simulink model "M_6DoF_BS_Full_backup_11_25_2018"  (R2018a)
settings: Solver=ode4  StartTime=0.0  StopTime=80  FixedStep=0.01  RelTol=1e-3  EnableMultiTasking=on
values from neighbouring files (symbols this model uses):
  b = 1.5652e-08 * (60/(2*pi))^2    (= 1.42729124973e-06)    [Main_run.m]    (also in golden_search.m = x2)
  cbar = 0.04    [Main_run.m]
  Cd = 0.001    [Main_run.m]
  deltaT = 15    [Main_run.m]
  g = 9.81    [Main_run.m]
  Gama1 = diag([3,3,3])    [Main_run.m]
  Gama2 = diag([0.1,0.1,0.1])    [Main_run.m]
  I_B = diag([Ix,Iy,Iz])    [Main_run.m]
  I_r = 3.357e-5    (= 3.357e-05)    [Main_run.m]
  InitialEulerAngles = [psi_i,theta_i,phi_i]    [Main_run.m]
  k = 2.0862e-10 * (60/(2*pi))^2    (= 1.90238627983e-08)    [Main_run.m]    (also in golden_search.m = 2)
  Kd = diag([2,2,2])    [Main_run.m]
  Ki = diag([0.01,0.01,0.01])    [Main_run.m]
  Kp = diag([1,1,1])    [Main_run.m]
  l = 0.225    [Main_run.m]    (also in try1.m = nb * trapz(psi, cl * 0.5 .* rho .* (vt*u).^2 .*c2 , 2) / (2*; try2.m = nb * trapz(psi, cl * 0.5 .* rho .* (vt*u).^2 .*c2 , 2) / (2*)
  Lambda = diag([10,10,10])    [Main_run.m]
  m = 1.035 * 4/6    (= 0.69)    [Main_run.m]
  Omega_i = [0;0;0]    [Main_run.m]
  r = linspace(floor(nr*0.01)/nr,1,nr)    [Main_run.m]    (also in Propeller.m = geometry(10,1:nr); try1.m = geometry(10,1:nr); try2.m = geometry(10,1:nr))
  R_i = [0.0;0.0;0.0]    [Main_run.m]
  t_phase3 = 10    [Main_run.m]
  Tbar = diag([15,15,15])    [Main_run.m]
  tf_phase1 = 10    [Main_run.m]
  tf_phase2 = tf_phase1 + length_phase2*60    (= 70)    [Main_run.m]
  V_i = [0.0;0.0;-0.001]    [Main_run.m]
  Wind_dir = 30 + 180    (= 210)    [Main_run.m]
  xdot_cruise = 15    [Main_run.m]
  zf_phase1 = -40    [Main_run.m]
undefined symbols (not defined in the file or in its folder): eul_0, HDBK, MIL, Moderate, wind_table, wind_time
libraries: sharedtransform x6, aerolibconvert2 x3, aerolibwind2 x3, sharedutil x2, simulink x1, aerolibutil x1, dspmathops x1
(part 1 of 2)
settings Model: SimulationMode=accelerator  Creator=EhsanTaheri  LastModifiedBy=behdad
settings SolverCC: AlgebraicLoopSolver=LineSearch
settings DataIOCC: LimitDataPoints=on  SaveFormat=Array
settings OptimizationCC: EfficientMapNaN2IntZero=off  LifeSpan=inf
settings DebuggingCC: SolverPrmCheckMsg=warning  SFUnexpectedBacktrackingDiag=warning  SFNoUnconditionalDefaultTransitionDiag=warning  SFExecutionAtInitializationDiag=none
settings HardwareCC: ProdBitPerPointer=32  ProdBitPerSizeT=32  ProdBitPerPtrDiffT=32  ProdLargestAtomicFloat=None  ProdIntDivRoundTo=Undefined  ProdEndianess=Unspecified  ProdWordSize=32  ProdHWDeviceType=32-bit Generic  TargetBitPerLong=64  TargetBitPerPointer=64  TargetBitPerSizeT=64  TargetBitPerPtrDiffT=64  TargetLongLongMode=on  TargetIntDivRoundTo=Zero  TargetEndianess=LittleEndian  TargetWordSize=64  TargetHWDeviceType=MATLAB Host  ProdEqTarget=off
settings ModelReferenceCC: PropagateSignalLabelsOutOfModel=off
settings CodeAppCC: MaxIdLength=128
settings GRTTargetCC: TargetLangStandard=C89/C90 (ANSI)  CombineOutputUpdateFcns=off  GRTInterface=on
settings ConfigComp: CovMetricSettings=dw  CovHtmlReporting=on  CovSaveCumulativeToWorkspaceVar=on  CovSaveSingleToWorkspaceVar=on  CovExternalEMLEnable=off  CovSFcnEnable=off

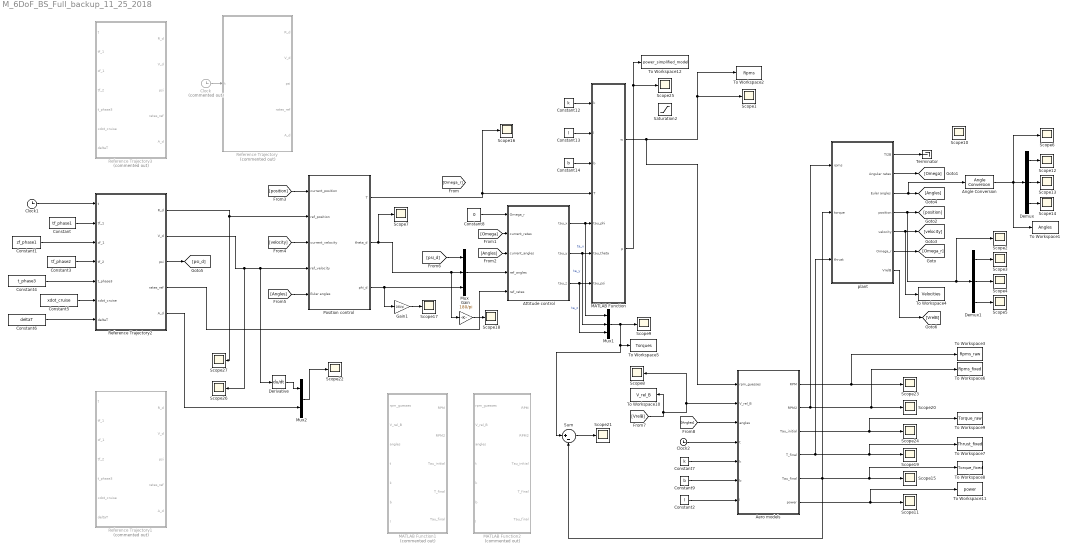
== system M_6DoF_BS_Full_backup_11_25_2018 ==
  Aero models : Subsystem
  Angle Conversion : aerolibconvert2/Angle Conversion  IU=rad  OU=deg
  Attitude control : Subsystem
  Clock : Clock  Commented=on
  Clock1 : Clock
  Clock2 : Clock
  Constant : Constant  Value=tf_phase1
  Constant1 : Constant  Value=zf_phase1
  Constant12 : Constant  Value=k
  Constant13 : Constant  Value=l
  Constant14 : Constant  Value=b
  Constant2 : Constant  Value=l
  Constant3 : Constant  Value=tf_phase2
  Constant4 : Constant  Value=t_phase3
  Constant5 : Constant  Value=xdot_cruise
  Constant6 : Constant  Value=deltaT
  Constant7 : Constant  Value=k
  Constant8 : Constant  Value=0
  Constant9 : Constant  Value=b
  Demux : Demux  Outputs=3
  Demux1 : Demux  Outputs=3
  Derivative : Derivative
  Gain : Gain  Gain=180/pi
  Gain1 : Gain  Gain=180/pi
  MATLAB Function : MATLAB Function  TreatAsAtomicUnit=on
  MATLAB Function1 : MATLAB Function  Commented=on  TreatAsAtomicUnit=on
  MATLAB Function2 : MATLAB Function  Commented=on  TreatAsAtomicUnit=on
  Mux : Mux  Inputs=3
  Mux1 : Mux  Inputs=3
  Mux2 : Mux  Inputs=2
  Position control : Subsystem
  Reference Trajectory : MATLAB Function  Commented=on  TreatAsAtomicUnit=on
  Reference Trajectory1 : MATLAB Function  Commented=on  TreatAsAtomicUnit=on
  Reference Trajectory2 : MATLAB Function  TreatAsAtomicUnit=on
  Reference Trajectory3 : MATLAB Function  Commented=on  TreatAsAtomicUnit=on
  Saturation2 : Saturate  UpperLimit=850  LowerLimit=200
  Scope{1..27} (27 alike) : Scope
  Sum : Sum  Inputs=|+-
  Terminator : Terminator
  To Workspace1 : ToWorkspace  VariableName=Angles  SampleTime=-1
  To Workspace10 : ToWorkspace  VariableName=V_rel_B  SampleTime=-1
  To Workspace11 : ToWorkspace  VariableName=power  SampleTime=-1
  To Workspace12 : ToWorkspace  VariableName=power_simplified_model  SampleTime=-1
  To Workspace2 : ToWorkspace  VariableName=Rpms  SampleTime=-1
  To Workspace3 : ToWorkspace  VariableName=Rpms_raw  SampleTime=-1
  To Workspace4 : ToWorkspace  VariableName=Velocities  SaveFormat=Structure With Time  SampleTime=-1
  To Workspace5 : ToWorkspace  VariableName=Torques  SampleTime=-1
  To Workspace6 : ToWorkspace  VariableName=Rpms_fixed  SampleTime=-1
  To Workspace7 : ToWorkspace  VariableName=Thrust_fixed  SampleTime=-1
  To Workspace8 : ToWorkspace  VariableName=Torque_fixed  SampleTime=-1
  To Workspace9 : ToWorkspace  VariableName=Torque_raw  SampleTime=-1
  plant : Subsystem
  wires:
  Demux/3 -> Scope14/1
  Demux/2 -> Scope13/1
  Demux/1 -> Scope12/1
  Demux1/3 -> Scope5/1
  Demux1/2 -> Scope4/1
  Demux1/1 -> Scope3/1
  Angle Conversion/1 -> Scope6/1, To Workspace1/1, Demux/1
  Constant12/1 -> MATLAB Function/1(k)
  Constant13/1 -> MATLAB Function/2(l)
  Constant14/1 -> MATLAB Function/3(b)
  plant/1(TI2B) -> Terminator/1
  plant/6(Omega_r) -> [Omega_r]
  plant/2(Angular rates) -> [Omega]
  [Omega] -> Attitude control/2(current_rates)
  plant/5(velocity) -> [velocity], To Workspace4/1
  [Angles] -> Attitude control/3(current_angles)
  Position control/1(T) -> Scope16/1, MATLAB Function/4(T)
  Attitude control/1(tau_x) -> Mux1/1, MATLAB Function/5(tau_phi)  "ta_x"
  Attitude control/2(tau_y) -> Mux1/2, MATLAB Function/6(tau_theta)  "ta_y"
  Attitude control/3(tau_z) -> Mux1/3, MATLAB Function/7(tau_psi)  "ta_z"
  [position] -> Position control/1(current_position)
  [velocity] -> Position control/3(current_velocity)
  Position control/2(theta_d) -> Scope7/1, Gain/1, Mux/2
  Position control/3(phi_d) -> Gain1/1, Mux/3
  Mux/1 -> Attitude control/4(ref_angles)
  plant/3(Euler angles) -> Angle Conversion/1, [Angles]
  Reference Trajectory2/3(psi) -> [psi_d]
  [psi_d] -> Mux/1
  Reference Trajectory2/1(R_d) -> Scope27/1, Position control/2(ref_position)
  [Angles] -> Position control/5(Euler angles)
  plant/4(position) -> [position], Scope2/1, Demux1/1
  Gain/1 -> Scope18/1
  Reference Trajectory2/5(A_d) -> Mux2/2
  Reference Trajectory2/2(V_d) -> Scope26/1, Derivative/1, Position control/4(ref_velocity)
  Derivative/1 -> Mux2/1
  Mux2/1 -> Scope22/1
  Gain1/1 -> Scope17/1
  Reference Trajectory2/4(rates_ref) -> Attitude control/5(ref_rates)
  Constant8/1 -> Attitude control/1(Omega_r)
  Clock/1 -> Reference Trajectory/1(t)
  Constant6/1 -> Reference Trajectory2/7(deltaT)
  Constant4/1 -> Reference Trajectory2/5(t_phase3)
  Clock1/1 -> Reference Trajectory2/1(t)
  Constant5/1 -> Reference Trajectory2/6(xdot_cruise)
  Constant1/1 -> Reference Trajectory2/3(zf_1)
  Constant3/1 -> Reference Trajectory2/4(tf_2)
  Constant/1 -> Reference Trajectory2/2(tf_1)
  MATLAB Function/1(w) -> Aero models/1(rpm_guesses), To Workspace2/1, Scope1/1
  Constant9/1 -> Aero models/6(b)
  Sum/1 -> Scope21/1
  [VrelB] -> Scope8/1, Aero models/2(V_rel_B), To Workspace10/1
  Constant7/1 -> Aero models/5(k)
  Constant2/1 -> Aero models/7(l)
  Mux1/1 -> Sum/1, To Workspace5/1, Scope9/1
  [Angles] -> Aero models/3(angles)
  Clock2/1 -> Aero models/4(t)
  Aero models/5(Tau_final) -> plant/2("torque "), To Workspace8/1, Scope15/1, Sum/2
  Aero models/3(Tau_initial) -> To Workspace9/1, Scope24/1
  Aero models/2(RPM2) -> Scope20/1, To Workspace6/1, plant/1(rpms)
  Aero models/1(RPM) -> Scope23/1, To Workspace3/1
  Aero models/4(T_final) -> plant/3(thrust), To Workspace7/1, Scope19/1
  plant/7(VrelB) -> [VrelB]
  Aero models/6(power) -> To Workspace11/1, Scope11/1
  MATLAB Function/2(p) -> Scope25/1, To Workspace12/1

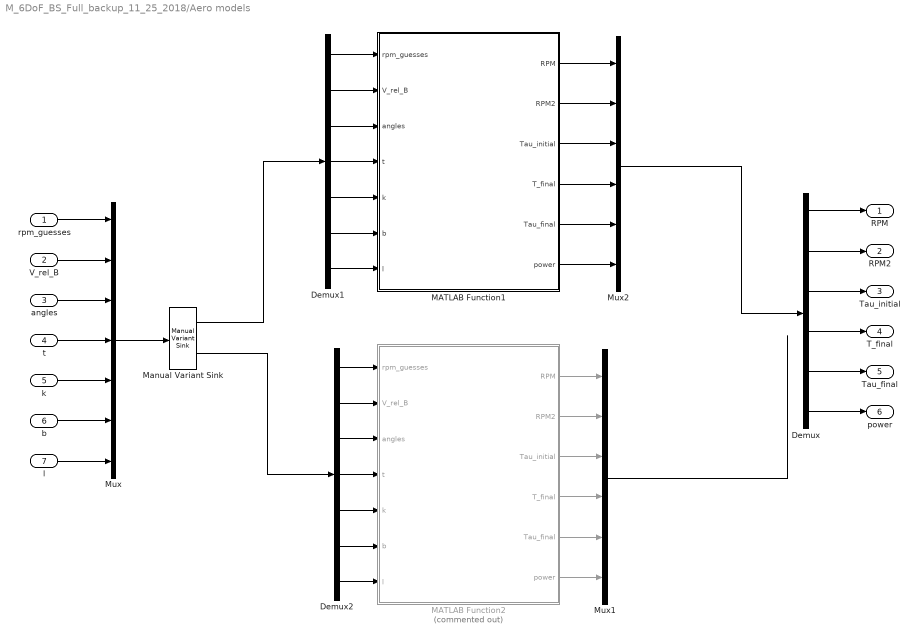
== system M_6DoF_BS_Full_backup_11_25_2018/Aero models ==
  rpm_guesses : Inport
  V_rel_B : Inport  Port=2
  angles : Inport  Port=3
  t : Inport  Port=4
  k : Inport  Port=5
  b : Inport  Port=6
  l : Inport  Port=7
  Demux : Demux  Outputs=[4 4 3 1 3 1]
  Demux1 : Demux  Outputs=[4 3 3 1 1 1 1]
  Demux2 : Demux  Outputs=[4 3 3 1 1 1 1]
  MATLAB Function1 : MATLAB Function  TreatAsAtomicUnit=on
  MATLAB Function2 : MATLAB Function  Commented=on  TreatAsAtomicUnit=on
  Manual Variant Sink : simulink/Signal Routing/Manual Variant Sink  NumChoices=2  OverrideUsingVariant=V_1
      settings: SourceProductName=Simulink
  Mux : Mux  Inputs=7
  Mux1 : Mux  Inputs=6
  Mux2 : Mux  Inputs=6
  RPM : Outport
  RPM2 : Outport  Port=2
  Tau_initial : Outport  Port=3
  T_final : Outport  Port=4
  Tau_final : Outport  Port=5
  power : Outport  Port=6
  wires:
  rpm_guesses/1 -> Mux/1
  V_rel_B/1 -> Mux/2
  angles/1 -> Mux/3
  t/1 -> Mux/4
  k/1 -> Mux/5
  b/1 -> Mux/6
  l/1 -> Mux/7
  Demux/3 -> Tau_initial/1
  Demux/4 -> T_final/1
  Demux/5 -> Tau_final/1
  Demux/2 -> RPM2/1
  Demux/1 -> RPM/1
  MATLAB Function2/5(Tau_final) -> Mux1/5
  MATLAB Function2/4(T_final) -> Mux1/4
  MATLAB Function2/3(Tau_initial) -> Mux1/3
  MATLAB Function2/2(RPM2) -> Mux1/2
  MATLAB Function2/1(RPM) -> Mux1/1
  MATLAB Function1/5(Tau_final) -> Mux2/5
  MATLAB Function1/4(T_final) -> Mux2/4
  MATLAB Function1/3(Tau_initial) -> Mux2/3
  MATLAB Function1/2(RPM2) -> Mux2/2
  MATLAB Function1/1(RPM) -> Mux2/1
  Demux1/7 -> MATLAB Function1/7(l)
  Demux1/6 -> MATLAB Function1/6(b)
  Demux1/5 -> MATLAB Function1/5(k)
  Demux1/4 -> MATLAB Function1/4(t)
  Demux1/3 -> MATLAB Function1/3(angles)
  Demux1/2 -> MATLAB Function1/2(V_rel_B)
  Demux1/1 -> MATLAB Function1/1(rpm_guesses)
  Demux2/7 -> MATLAB Function2/7(l)
  Demux2/6 -> MATLAB Function2/6(b)
  Demux2/5 -> MATLAB Function2/5(k)
  Demux2/4 -> MATLAB Function2/4(t)
  Demux2/3 -> MATLAB Function2/3(angles)
  Demux2/2 -> MATLAB Function2/2(V_rel_B)
  Demux2/1 -> MATLAB Function2/1(rpm_guesses)
  Mux/1 -> Manual Variant Sink/1
  Manual Variant Sink/1 -> Demux1/1
  Manual Variant Sink/2 -> Demux2/1
  MATLAB Function2/6(power) -> Mux1/6
  Demux/6 -> power/1
  MATLAB Function1/6(power) -> Mux2/6
  Mux1/1 -> ?
  Mux2/1 -> Demux/1

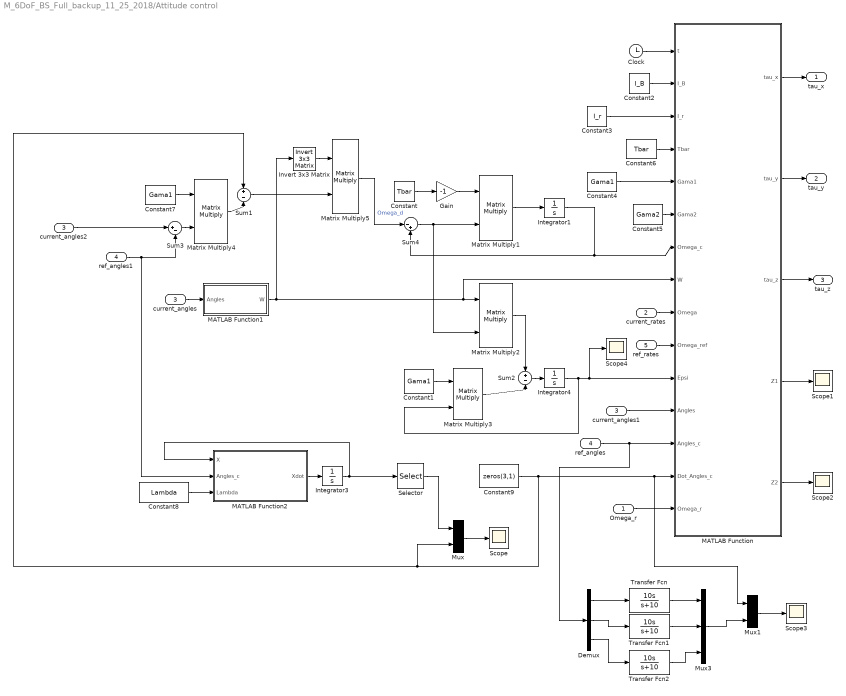
== system M_6DoF_BS_Full_backup_11_25_2018/Attitude control ==
  Omega_r : Inport
  current_rates : Inport  Port=2
  current_angles : Inport  Port=3
  ref_angles : Inport  Port=4
  ref_rates : Inport  Port=5
  Clock : Clock
  Constant : Constant  Value=Tbar
  Constant1 : Constant  Value=Gama1
  Constant2 : Constant  Value=I_B
  Constant3 : Constant  Value=I_r
  Constant4 : Constant  Value=Gama1
  Constant5 : Constant  Value=Gama2
  Constant6 : Constant  Value=Tbar
  Constant7 : Constant  Value=Gama1
  Constant8 : Constant  Value=Lambda
  Constant9 : Constant  Value=zeros(3,1)
  Demux : Demux  Outputs=3
  Gain : Gain  Gain=-1
  Integrator1 : Integrator  InitialCondition=zeros(3,1)
  Integrator3 : Integrator  InitialCondition=[InitialEulerAngles';zeros(3,1)]
  Integrator4 : Integrator  InitialCondition=zeros(3,1)
  Invert 3x3 Matrix : aerolibutil/Invert  3x3 Matrix
  MATLAB Function : MATLAB Function  TreatAsAtomicUnit=on
  MATLAB Function1 : MATLAB Function  TreatAsAtomicUnit=on
  MATLAB Function2 : MATLAB Function  TreatAsAtomicUnit=on
  Matrix Multiply{1..5} (5 alike) : Product  Multiplication=Matrix(*)
  Mux : Mux  Inputs=2
  Mux1 : Mux  Inputs=2
  Mux3 : Mux  Inputs=3
  Scope{,1..4} (5 alike) : Scope
  Selector : Selector  InputPortWidth=6  IndexOptions=Index vector (dialog)  Indices=[4 5 6]  OutputSizes=1
  Sum1 : Sum  Inputs=+|-
  Sum2 : Sum  Inputs=+|-
  Sum3 : Sum  Inputs=|+-
  Sum4 : Sum  Inputs=|-+
  Transfer Fcn : TransferFcn  Numerator=[10 0]  Denominator=[1 10]
  Transfer Fcn1 : TransferFcn  Numerator=[10 0]  Denominator=[1 10]
  Transfer Fcn2 : TransferFcn  Numerator=[10 0]  Denominator=[1 10]
  current_angles1 : InportShadow  Port=3
  current_angles2 : InportShadow  Port=3
  ref_angles1 : InportShadow  Port=4
  tau_x : Outport
  tau_y : Outport  Port=2
  tau_z : Outport  Port=3
  wires:
  Omega_r/1 -> MATLAB Function/15(Omega_r)
  MATLAB Function/1(tau_x) -> tau_x/1
  MATLAB Function/2(tau_y) -> tau_y/1
  MATLAB Function/3(tau_z) -> tau_z/1
  Matrix Multiply5/1 -> Sum4/1  "Omega_d"
  Gain/1 -> Matrix Multiply1/1
  Constant/1 -> Gain/1
  current_angles/1 -> MATLAB Function1/1(Angles)
  MATLAB Function1/1(W) -> Invert 3x3 Matrix/1, MATLAB Function/8(W), Matrix Multiply2/1
  Matrix Multiply1/1 -> Integrator1/1
  Matrix Multiply2/1 -> Sum2/1
  Matrix Multiply3/1 -> Sum2/2
  Constant1/1 -> Matrix Multiply3/1
  Integrator4/1 -> Matrix Multiply3/2, Scope4/1, MATLAB Function/11(Epsi)
  current_rates/1 -> MATLAB Function/9(Omega)
  current_angles1/1 -> MATLAB Function/12(Angles)
  ref_angles/1 -> Demux/1, MATLAB Function/13(Angles_c)
  Constant4/1 -> MATLAB Function/5(Gama1)
  Constant5/1 -> MATLAB Function/6(Gama2)
  Constant6/1 -> MATLAB Function/4(Tbar)
  Constant2/1 -> MATLAB Function/2(I_B)
  Constant3/1 -> MATLAB Function/3(I_r)
  Constant7/1 -> Matrix Multiply4/1
  Sum3/1 -> Matrix Multiply4/2
  current_angles2/1 -> Sum3/1
  ref_angles1/1 -> MATLAB Function2/2(Angles_c), Sum3/2
  Matrix Multiply4/1 -> Sum1/2
  Invert 3x3 Matrix/1 -> Matrix Multiply5/1
  Sum1/1 -> Matrix Multiply5/2
  Integrator1/1 -> Sum4/2, MATLAB Function/7(Omega_c)
  Sum4/1 -> Matrix Multiply2/2, Matrix Multiply1/2
  Clock/1 -> MATLAB Function/1(t)
  MATLAB Function2/1(Xdot) -> Integrator3/1
  Integrator3/1 -> Selector/1, MATLAB Function2/1(X)
  Constant8/1 -> MATLAB Function2/3(Lambda)
  ref_rates/1 -> MATLAB Function/10(Omega_ref)
  Constant9/1 -> Mux/2, Sum1/1, Mux1/1, MATLAB Function/14(Dot_Angles_c)
  Selector/1 -> Mux/1
  MATLAB Function/4(Z1) -> Scope1/1
  MATLAB Function/5(Z2) -> Scope2/1
  Demux/1 -> Transfer Fcn/1
  Demux/2 -> Transfer Fcn1/1
  Demux/3 -> Transfer Fcn2/1
  Transfer Fcn1/1 -> Mux3/2
  Mux3/1 -> Mux1/2
  Mux1/1 -> Scope3/1
  Mux/1 -> Scope/1
  Sum2/1 -> Integrator4/1
  Transfer Fcn/1 -> Mux3/1
  Transfer Fcn2/1 -> Mux3/3

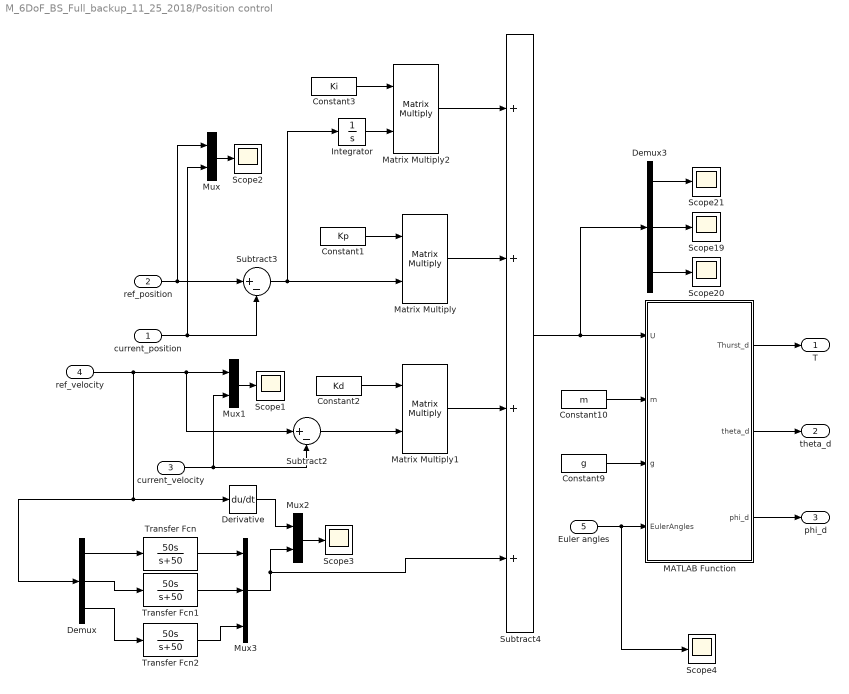
== system M_6DoF_BS_Full_backup_11_25_2018/Position control ==
  current_position : Inport
  ref_position : Inport  Port=2
  current_velocity : Inport  Port=3
  ref_velocity : Inport  Port=4
  Euler angles : Inport  Port=5
  Constant1 : Constant  Value=Kp
  Constant10 : Constant  Value=m
  Constant2 : Constant  Value=Kd
  Constant3 : Constant  Value=Ki
  Constant9 : Constant  Value=g
  Demux : Demux  Outputs=3
  Demux3 : Demux  Outputs=3
  Derivative : Derivative
  Integrator : Integrator  InitialCondition=zeros(3,1)
  MATLAB Function : MATLAB Function  TreatAsAtomicUnit=on
  Matrix Multiply : Product  Multiplication=Matrix(*)
  Matrix Multiply1 : Product  Multiplication=Matrix(*)
  Matrix Multiply2 : Product  Multiplication=Matrix(*)
  Mux : Mux  Inputs=2
  Mux1 : Mux  Inputs=2
  Mux2 : Mux  Inputs=2
  Mux3 : Mux  Inputs=3
  Scope{1..4,19..21} (7 alike) : Scope
  Subtract2 : Sum  Inputs=|+-
  Subtract3 : Sum  Inputs=|+-
  Subtract4 : Sum  Inputs=++++
  Transfer Fcn : TransferFcn  Numerator=[50 0]  Denominator=[1 50]
  Transfer Fcn1 : TransferFcn  Numerator=[50 0]  Denominator=[1 50]
  Transfer Fcn2 : TransferFcn  Numerator=[50 0]  Denominator=[1 50]
  T : Outport
  theta_d : Outport  Port=2
  phi_d : Outport  Port=3
  wires:
  MATLAB Function/2(theta_d) -> theta_d/1
  MATLAB Function/3(phi_d) -> phi_d/1
  MATLAB Function/1(Thurst_d) -> T/1
  Constant10/1 -> MATLAB Function/2(m)
  Constant9/1 -> MATLAB Function/3(g)
  ref_position/1 -> Subtract3/1, Mux/1
  current_position/1 -> Subtract3/2, Mux/2
  Subtract3/1 -> Matrix Multiply/2, Integrator/1
  Constant1/1 -> Matrix Multiply/1
  Subtract2/1 -> Matrix Multiply1/2
  Constant2/1 -> Matrix Multiply1/1
  Subtract4/1 -> Demux3/1, MATLAB Function/1(U)
  Euler angles/1 -> Scope4/1, MATLAB Function/4(EulerAngles)
  Mux/1 -> Scope2/1
  Mux1/1 -> Scope1/1
  Derivative/1 -> Mux2/1
  Mux2/1 -> Scope3/1
  Demux/1 -> Transfer Fcn/1
  Demux/2 -> Transfer Fcn1/1
  Demux/3 -> Transfer Fcn2/1
  Transfer Fcn1/1 -> Mux3/2
  Mux3/1 -> Subtract4/4, Mux2/2
  Integrator/1 -> Matrix Multiply2/2
  Constant3/1 -> Matrix Multiply2/1
  Matrix Multiply1/1 -> Subtract4/3
  Matrix Multiply/1 -> Subtract4/2
  Matrix Multiply2/1 -> Subtract4/1
  Transfer Fcn/1 -> Mux3/1
  Transfer Fcn2/1 -> Mux3/3
  current_velocity/1 -> Subtract2/2, Mux1/2
  Demux3/3 -> Scope20/1
  Demux3/1 -> Scope21/1
  Demux3/2 -> Scope19/1
  ref_velocity/1 -> Derivative/1, Demux/1, Mux1/1, Subtract2/1

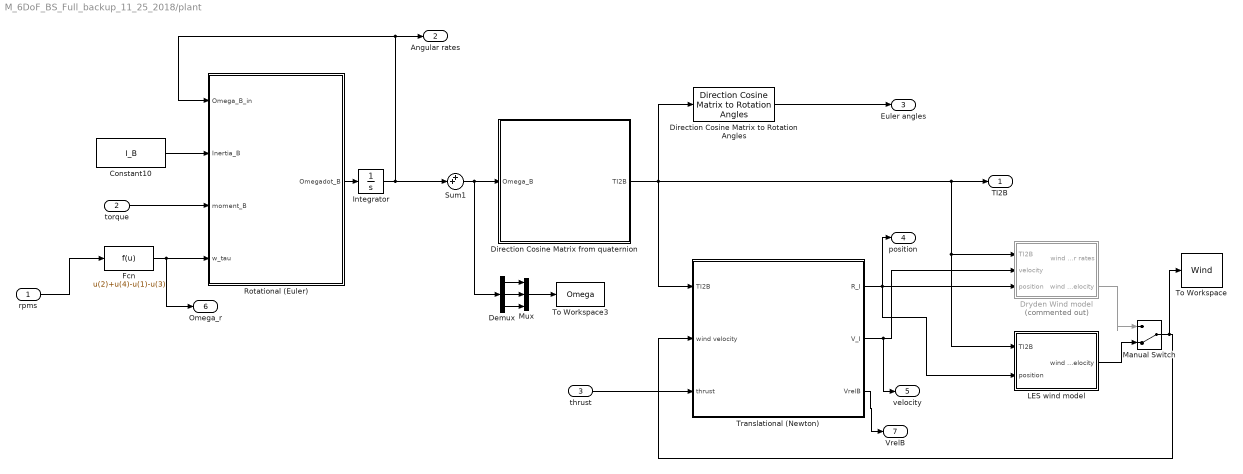
== system M_6DoF_BS_Full_backup_11_25_2018/plant ==
  rpms : Inport
  "torque " : Inport  Port=2
  thrust : Inport  Port=3
  Constant10 : Constant  Value=I_B
  Demux : Demux  Outputs=3
  Direction Cosine Matrix to Rotation Angles : sharedtransform/Direction Cosine Matrix to Rotation Angles  rotationOrder=ZYX  aMode=aMode  action=None  tolerance=eps(2)
      settings: SourceProductName=Aerospace Blockset  SourceProductBaseCode=AE
  Direction Cosine Matrix from quaternion : Subsystem
  Dryden Wind model : Subsystem  Commented=on
  Fcn : Fcn  Expr=u(2)+u(4)-u(1)-u(3)
  Integrator : Integrator  InitialCondition=Omega_i
  LES wind model : Subsystem
  Manual Switch : ManualSwitch  CurrentSetting=0
  Mux : Mux  Inputs=3
  Rotational (Euler) : Subsystem
  Sum1 : Sum  Inputs=++|
  To Workspace : ToWorkspace  VariableName=Wind  SampleTime=-1
      settings: Save2DSignal=2-D array (concatenate along first dimension)
  To Workspace3 : ToWorkspace  VariableName=Omega  SampleTime=-1
  Translational (Newton) : Subsystem
  TI2B : Outport
  Angular rates : Outport  Port=2
  Euler angles : Outport  Port=3
  position : Outport  Port=4
  velocity : Outport  Port=5
  Omega_r : Outport  Port=6
  VrelB : Outport  Port=7
  wires:
  Translational (Newton)/2(V_I) -> velocity/1, Dryden Wind model/2(velocity)
  Direction Cosine Matrix to Rotation Angles/1 -> Euler angles/1
  Constant10/1 -> Rotational (Euler)/2(Inertia_B)
  Rotational (Euler)/1(Omegadot_B) -> Integrator/1
  Direction Cosine Matrix from quaternion/1(TI2B) -> Translational (Newton)/1(TI2B), LES wind model/1(TI2B), Dryden Wind model/1(TI2B), TI2B/1, Direction Cosine Matrix to Rotation Angles/1
  rpms/1 -> Fcn/1
  Fcn/1 -> Rotational (Euler)/4(w_tau), Omega_r/1
  Integrator/1 -> Sum1/2, Angular rates/1, Rotational (Euler)/1(Omega_B_in)
  Sum1/1 -> Demux/1, Direction Cosine Matrix from quaternion/1(Omega_B)
  Demux/1 -> Mux/1
  Demux/2 -> Mux/2
  Demux/3 -> Mux/3
  Mux/1 -> To Workspace3/1
  thrust/1 -> Translational (Newton)/3(thrust)
  "torque "/1 -> Rotational (Euler)/3(moment_B)
  Translational (Newton)/3(VrelB) -> VrelB/1
  Translational (Newton)/1(R_I) -> Dryden Wind model/3(position), LES wind model/2(position), position/1
  LES wind model/1(wind velocity) -> Manual Switch/2
  Dryden Wind model/2(wind velocity) -> Manual Switch/1
  Manual Switch/1 -> To Workspace/1, Translational (Newton)/2(wind velocity)

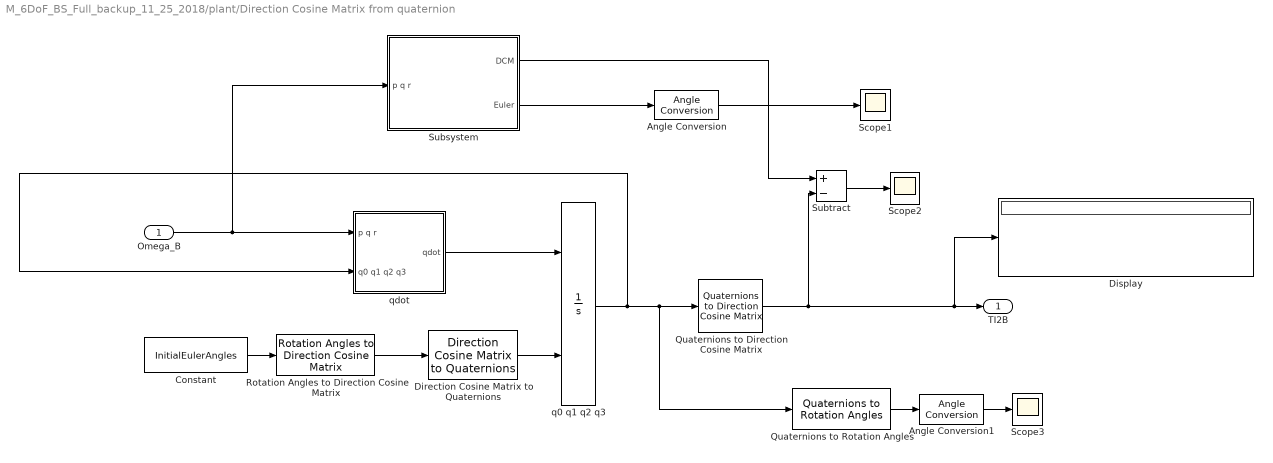
== system M_6DoF_BS_Full_backup_11_25_2018/plant/Direction Cosine Matrix from quaternion ==
  Omega_B : Inport
  Angle Conversion : aerolibconvert2/Angle Conversion  IU=rad  OU=deg
  Angle Conversion1 : aerolibconvert2/Angle Conversion  IU=rad  OU=deg
  Constant : Constant  Value=InitialEulerAngles
  Direction Cosine Matrix to Quaternions : sharedtransform/Direction Cosine Matrix  to Quaternions  aMode=aMode  action=None  tolerance=eps(2)
      settings: SourceProductName=Aerospace Blockset  SourceProductBaseCode=AE
  Display : Display
  Quaternions to Direction Cosine Matrix : sharedtransform/Quaternions to  Direction Cosine Matrix  aMode=aMode
      settings: SourceProductName=Aerospace Blockset  SourceProductBaseCode=AE
  Quaternions to Rotation Angles : sharedtransform/Quaternions to Rotation Angles  rotationOrder=ZYX  aMode=aMode
      settings: SourceProductBaseCode=AE
  Rotation Angles to Direction Cosine Matrix : sharedtransform/Rotation Angles to Direction Cosine Matrix  rotationOrder=ZYX  aMode=aMode
      settings: SourceProductBaseCode=AE
  Scope1 : Scope
  Scope2 : Scope
  Scope3 : Scope
  Subsystem : Subsystem
  Subtract : Sum  Inputs=+-
  q0 q1 q2 q3 : Integrator  InitialConditionSource=external
  qdot : Subsystem
  TI2B : Outport
  wires:
  Direction Cosine Matrix to Quaternions/1 -> q0 q1 q2 q3/2
  Omega_B/1 -> qdot/1(p q r), Subsystem/1("p q r ")
  q0 q1 q2 q3/1 -> Quaternions to Rotation Angles/1, Quaternions to Direction Cosine Matrix/1, qdot/2(q0 q1 q2 q3)
  qdot/1(qdot) -> q0 q1 q2 q3/1
  Rotation Angles to Direction Cosine Matrix/1 -> Direction Cosine Matrix to Quaternions/1
  Constant/1 -> Rotation Angles to Direction Cosine Matrix/1
  Subsystem/2(Euler) -> Angle Conversion/1
  Angle Conversion/1 -> Scope1/1
  Quaternions to Direction Cosine Matrix/1 -> Subtract/2, Display/1, TI2B/1
  Subsystem/1(DCM) -> Subtract/1
  Subtract/1 -> Scope2/1
  Quaternions to Rotation Angles/1 -> Angle Conversion1/1
  Angle Conversion1/1 -> Scope3/1

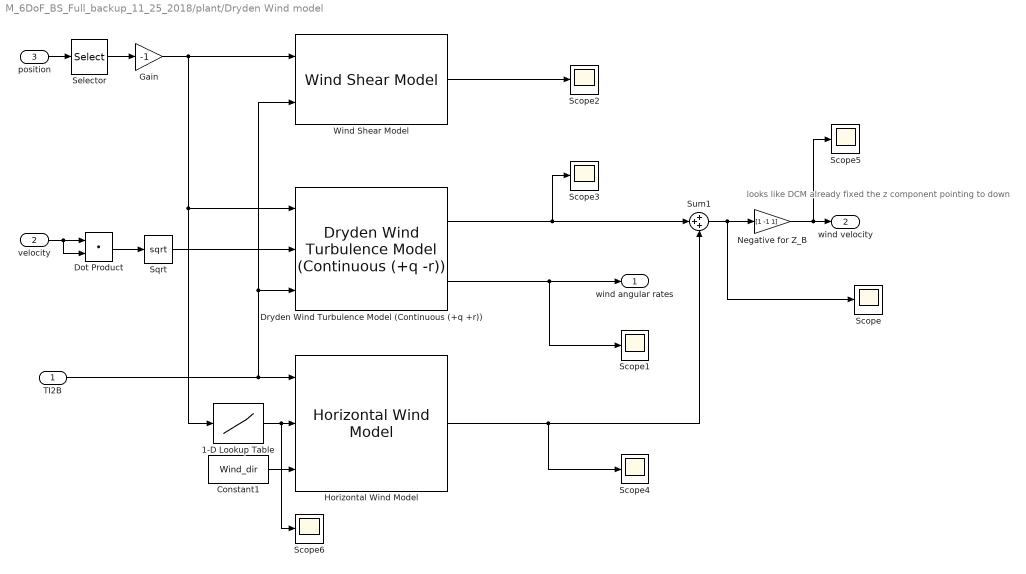
== system M_6DoF_BS_Full_backup_11_25_2018/plant/Dryden Wind model ==
  note: looks like DCM already fixed the z component pointing to down
  TI2B : Inport
  velocity : Inport  Port=2
  position : Inport  Port=3
  1-D Lookup Table : Lookup_n-D  NumberOfTableDimensions=1  BreakpointsSpecification=Even spacing  BreakpointsForDimension1=[-5:5]  BreakpointsForDimension1FirstPoint=0  BreakpointsForDimension1Spacing=2  Table=wind_table  InternalRulePriority=Speed  RndMeth=Simplest  InputSameDT=on
  Constant1 : Constant  Value=Wind_dir
  Dot Product : DotProduct  InputSameDT=on  OutDataTypeStr=Inherit: Inherit via internal rule
  Dryden Wind Turbulence Model (Continuous (+q +r)) : aerolibwind2/Dryden Wind Turbulence Model  (Continuous (+q -r))  units=Metric (MKS)  spec=MIL-HDBK-1797B  model=Continuous Dryden (+q +r)  W20=V_wind_at6m  Wdeg=Angle_wind_at6m  TurbProb=10^-3 - Moderate  L_high=533.4  Wingspan=2  ts=0.01  Seed=[23341 23342 23343 23344]  T_on=on
      settings: SourceProductName=Aerospace Blockset
  Gain : Gain  Gain=-1
  Horizontal Wind Model : aerolibwind2/Horizontal Wind Model  units=Metric (MKS)  Vw_source=External  Vwind=5  W_source=External  Wdeg=0
      settings: SourceProductName=Aerospace Blockset  SourceProductBaseCode=AE
  Negative for Z_B : Gain  Gain=[1 -1 1]
  Scope{,1..6} (7 alike) : Scope
  Selector : Selector  InputPortWidth=3  IndexOptions=Index vector (dialog)  Indices=[3]  OutputSizes=1
  Sqrt : Sqrt  SaturateOnIntegerOverflow=on
  Sum1 : Sum  Inputs=+++
  Wind Shear Model : aerolibwind2/Wind Shear Model  units=Metric (MKS)  phase=Other  W_20=V_wind_at6m  Wdeg=Angle_wind_at6m
      settings: SourceProductName=Aerospace Blockset
  wind angular rates : Outport
  wind velocity : Outport  Port=2
  wires:
  Gain/1 -> 1-D Lookup Table/1, Dryden Wind Turbulence Model (Continuous (+q +r))/1, Wind Shear Model/1
  Dryden Wind Turbulence Model (Continuous (+q +r))/2 -> wind angular rates/1, Scope1/1
  Sqrt/1 -> Dryden Wind Turbulence Model (Continuous (+q +r))/2
  Dryden Wind Turbulence Model (Continuous (+q +r))/1 -> Scope3/1, Sum1/2
  Sum1/1 -> Negative for Z_B/1, Scope/1
  Constant1/1 -> Horizontal Wind Model/3
  Horizontal Wind Model/1 -> Sum1/3, Scope4/1
  velocity/1 -> Dot Product/2, Dot Product/1
  Dot Product/1 -> Sqrt/1
  TI2B/1 -> Wind Shear Model/2, Dryden Wind Turbulence Model (Continuous (+q +r))/3, Horizontal Wind Model/1
  position/1 -> Selector/1
  Wind Shear Model/1 -> Scope2/1
  Selector/1 -> Gain/1
  Negative for Z_B/1 -> Scope5/1, wind velocity/1
  1-D Lookup Table/1 -> Scope6/1, Horizontal Wind Model/2

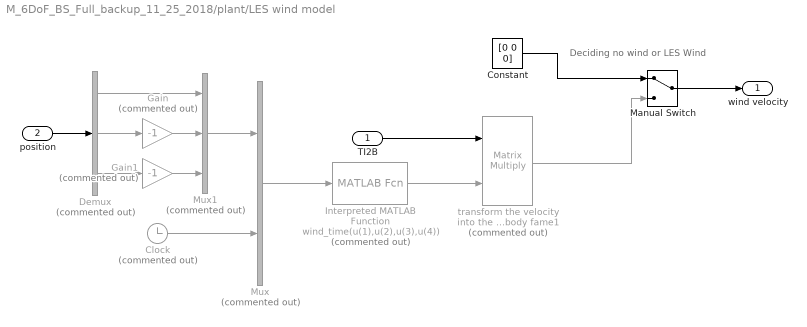
== system M_6DoF_BS_Full_backup_11_25_2018/plant/LES wind model ==
  note: Deciding no wind or LES Wind
  TI2B : Inport
  position : Inport  Port=2
  Clock : Clock  Commented=on
  Constant : Constant  Value=[0 0 0]
  Demux : Demux  Commented=on  Outputs=3
  Gain : Gain  Commented=on  Gain=-1
  Gain1 : Gain  Commented=on  Gain=-1
  Interpreted MATLAB Function : MATLABFcn  Commented=on  MATLABFcn=wind_time(u(1),u(2),u(3),u(4))
  Manual Switch : ManualSwitch
  Mux : Mux  Commented=on  Inputs=2
  Mux1 : Mux  Commented=on  Inputs=3
  transform the velocity into the body fame1 : Product  Commented=on  Multiplication=Matrix(*)
  wind velocity : Outport
  wires:
  Gain/1 -> Mux1/2
  Clock/1 -> Mux/2
  Gain1/1 -> Mux1/3
  Mux1/1 -> Mux/1
  Demux/3 -> Gain1/1
  Demux/1 -> Mux1/1
  position/1 -> Demux/1
  Demux/2 -> Gain/1
  Mux/1 -> Interpreted MATLAB Function/1
  TI2B/1 -> transform the velocity into the body fame1/1
  Interpreted MATLAB Function/1 -> transform the velocity into the body fame1/2
  Constant/1 -> Manual Switch/1
  Manual Switch/1 -> wind velocity/1
  transform the velocity into the body fame1/1 -> Manual Switch/2

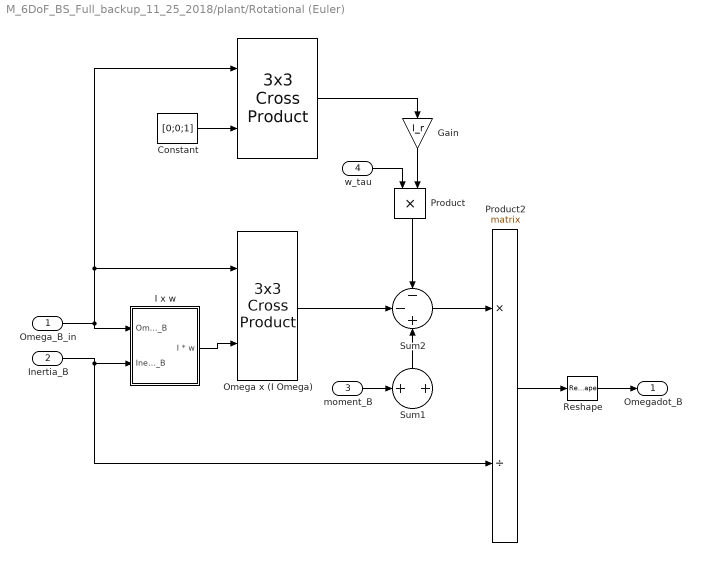
== system M_6DoF_BS_Full_backup_11_25_2018/plant/Rotational (Euler) ==
  Omega_B_in : Inport
  Inertia_B : Inport  Port=2
  moment_B : Inport  Port=3
  w_tau : Inport  Port=4
  " " : sharedutil/3x3 Cross Product  aMode=aMode
      settings: SourceProductBaseCode=AE
  Constant : Constant  Value=[0;0;1]
  Gain : Gain  Gain=I_r
  I x w : Subsystem
  Omega x (I Omega) : sharedutil/3x3 Cross Product  aMode=aMode
      settings: SourceProductBaseCode=AE
  Product : Product
  Product2 : Product  Inputs=*/  Multiplication=Matrix(*)  SaturateOnIntegerOverflow=on  OutDataTypeStr=Inherit: Same as first input
  Reshape : Reshape  OutputDimensionality=Column vector (2-D)
  Sum1 : Sum  SaturateOnIntegerOverflow=on
  Sum2 : Sum  Inputs=--+  SaturateOnIntegerOverflow=on
  Omegadot_B : Outport
  wires:
  Omega x (I Omega)/1 -> Sum2/2
  Omega_B_in/1 -> I x w/1(Omega_B), " "/1, Omega x (I Omega)/1
  Product2/1 -> Reshape/1
  Sum2/1 -> Product2/1
  I x w/1(I * w) -> Omega x (I Omega)/2
  Reshape/1 -> Omegadot_B/1
  Inertia_B/1 -> Product2/2, I x w/2(Inertia_B)
  Constant/1 -> " "/2
  " "/1 -> Gain/1
  Gain/1 -> Product/2
  w_tau/1 -> Product/1
  Product/1 -> Sum2/1
  moment_B/1 -> Sum1/1
  Sum1/1 -> Sum2/3

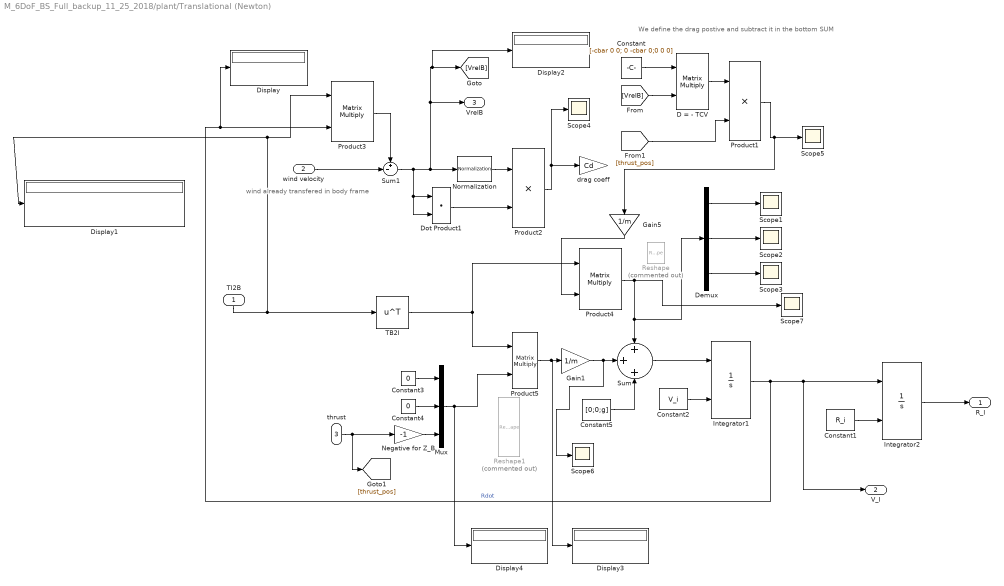
== system M_6DoF_BS_Full_backup_11_25_2018/plant/Translational (Newton) ==
  note: We define the drag postive and subtract it in the bottom SUM
  note: wind already transfered in body frame
  TI2B : Inport
  wind velocity : Inport  Port=2
  thrust : Inport  Port=3
  Constant : Constant  Value=[-cbar 0 0; 0 -cbar 0;0 0 0]
  Constant1 : Constant  Value=R_i
  Constant2 : Constant  Value=V_i
  Constant3 : Constant  Value=0
  Constant4 : Constant  Value=0
  Constant5 : Constant  Value=[0;0;g]
  D = - TCV : Product  Multiplication=Matrix(*)
  Demux : Demux  Outputs=3
  Display{,1..4} (5 alike) : Display
  Dot Product1 : DotProduct  InputSameDT=on  OutDataTypeStr=Inherit: Inherit via internal rule
  Gain1 : Gain  Gain=1/m
  Gain5 : Gain  Gain=1/m
  Integrator1 : Integrator  InitialConditionSource=external
  Integrator2 : Integrator  InitialConditionSource=external
  Mux : Mux  Inputs=3
  Negative for Z_B : Gain  Gain=-1
  Normalization : dspmathops/Normalization  NormType=2-norm  Bias=1e-10  NormOver=Each column  Dimension=1  roundingMode=Floor  overflowMode=off  accumDataTypeStr=Inherit: Same as product output  accumLastDataTypeStr=Inherit: Same as product output  outputDataTypeStr=Inherit: Same as product output  outputMin=[]  outputMax=[]  outputLastDataTypeStr=Inherit: Same as product output
      settings: SourceProductName=DSP System Toolbox
  Product1 : Product
  Product2 : Product
  Product3 : Product  Multiplication=Matrix(*)
  Product4 : Product  Multiplication=Matrix(*)
  Product5 : Product  Multiplication=Matrix(*)
  Reshape : Reshape  Commented=on
  Reshape1 : Reshape  Commented=on
  Scope{1..7} (7 alike) : Scope
  Sum : Sum  Inputs=+++
  Sum1 : Sum  Inputs=+-|
  TB2I : Math  Operator=transpose  SaturateOnIntegerOverflow=on
  drag coeff : Gain  Gain=Cd
  R_I : Outport
  V_I : Outport  Port=2
  VrelB : Outport  Port=3
  wires:
  Integrator1/1 -> V_I/1, Integrator2/1, Display/1, Product3/2  "Rdot"
  Constant2/1 -> Integrator1/2
  Constant1/1 -> Integrator2/2
  thrust/1 -> [thrust_pos], Negative for Z_B/1
  Constant3/1 -> Mux/1
  Constant4/1 -> Mux/2
  Mux/1 -> Display4/1, Product5/2
  Product5/1 -> Display3/1, Gain1/1
  Gain1/1 -> Scope6/1, Sum/2
  Constant5/1 -> Sum/3
  Sum/1 -> Integrator1/1
  Integrator2/1 -> R_I/1
  Negative for Z_B/1 -> Mux/3
  Product3/1 -> Sum1/1
  Dot Product1/1 -> Product2/2
  Product2/1 -> drag coeff/1, Scope4/1
  Gain5/1 -> Product4/2
  Normalization/1 -> Product2/1
  Product4/1 -> Sum/1, Demux/1, Scope7/1
  Demux/1 -> Scope1/1
  Demux/2 -> Scope2/1
  Demux/3 -> Scope3/1
  Sum1/1 -> VrelB/1, Display2/1, [VrelB], Normalization/1, Dot Product1/2, Dot Product1/1
  wind velocity/1 -> Sum1/2
  [thrust_pos] -> Product1/2
  Constant/1 -> D = - TCV/1
  D = - TCV/1 -> Product1/1
  Product1/1 -> Gain5/1, Scope5/1
  [VrelB] -> D = - TCV/2
  TI2B/1 -> TB2I/1, Product3/1, Display1/1
  TB2I/1 -> Product4/1, Product5/1

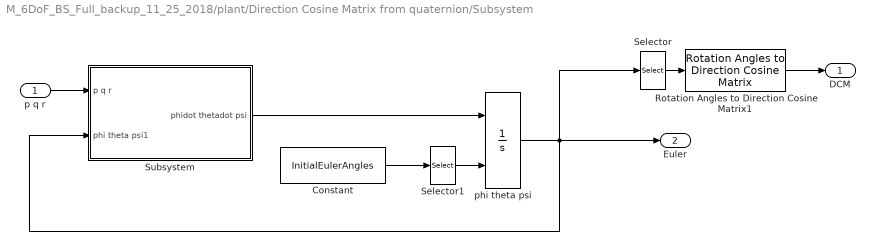
== system M_6DoF_BS_Full_backup_11_25_2018/plant/Direction Cosine Matrix from quaternion/Subsystem ==
  "p q r " : Inport
  Constant : Constant  Value=InitialEulerAngles
  Rotation Angles to Direction Cosine Matrix1 : sharedtransform/Rotation Angles to Direction Cosine Matrix  rotationOrder=ZYX  aMode=aMode
      settings: SourceProductBaseCode=AE
  Selector : Selector  InputPortWidth=3  IndexOptions=Index vector (dialog)  Indices=[3 2 1]  OutputSizes=1
  Selector1 : Selector  InputPortWidth=3  IndexOptions=Index vector (dialog)  Indices=[3 2 1]  OutputSizes=1
  Subsystem : Subsystem
  phi theta psi : Integrator  InitialConditionSource=external  InitialCondition=eul_0
  DCM : Outport
  Euler : Outport  Port=2
  wires:
  Subsystem/1(phidot thetadot psi) -> phi theta psi/1
  phi theta psi/1 -> Selector/1, Euler/1, Subsystem/2(phi theta psi1)
  Rotation Angles to Direction Cosine Matrix1/1 -> DCM/1
  Selector/1 -> Rotation Angles to Direction Cosine Matrix1/1
  "p q r "/1 -> Subsystem/1(p q r)
  Selector1/1 -> phi theta psi/2
  Constant/1 -> Selector1/1

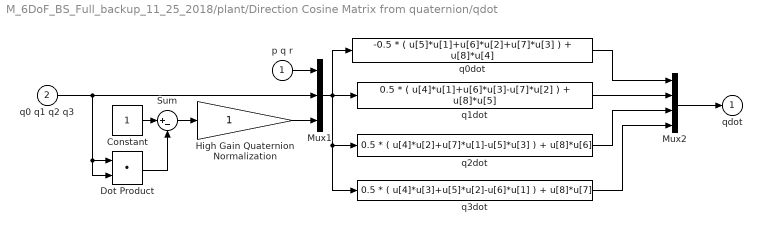
== system M_6DoF_BS_Full_backup_11_25_2018/plant/Direction Cosine Matrix from quaternion/qdot ==
  p q r : Inport
  q0 q1 q2 q3 : Inport  Port=2
  Constant : Constant
  Dot Product : DotProduct  OutDataTypeStr=Inherit: Inherit via internal rule
  High Gain Quaternion Normalization : Gain  SaturateOnIntegerOverflow=on  OutDataTypeStr=Inherit: Same as input  ParamDataTypeStr=Inherit: Same as input
  Mux1 : Mux  Inputs=[3 4 1]
  Mux2 : Mux
  Sum : Sum  Inputs=|+-  SaturateOnIntegerOverflow=on  InputSameDT=on  OutDataTypeStr=Inherit: Same as first input
  q0dot : Fcn  Expr=-0.5 * ( u[5]*u[1]+u[6]*u[2]+u[7]*u[3] ) + u[8]*u[4]
  q1dot : Fcn  Expr=0.5 * ( u[4]*u[1]+u[6]*u[3]-u[7]*u[2] ) + u[8]*u[5]
  q2dot : Fcn  Expr=0.5 * ( u[4]*u[2]+u[7]*u[1]-u[5]*u[3] ) + u[8]*u[6]
  q3dot : Fcn  Expr=0.5 * ( u[4]*u[3]+u[5]*u[2]-u[6]*u[1] ) + u[8]*u[7]
  qdot : Outport  InitialOutput=0
  wires:
  p q r/1 -> Mux1/1
  Dot Product/1 -> Sum/2
  High Gain Quaternion Normalization/1 -> Mux1/3
  Sum/1 -> High Gain Quaternion Normalization/1
  Constant/1 -> Sum/1
  Mux2/1 -> qdot/1
  q0dot/1 -> Mux2/1
  q1dot/1 -> Mux2/2
  q2dot/1 -> Mux2/3
  Mux1/1 -> q2dot/1, q3dot/1, q0dot/1, q1dot/1
  q3dot/1 -> Mux2/4
  q0 q1 q2 q3/1 -> Dot Product/1, Dot Product/2, Mux1/2

== system M_6DoF_BS_Full_backup_11_25_2018/plant/Rotational (Euler)/I x w ==
  Omega_B : Inport
  Inertia_B : Inport  Port=2
  Product : Product  Multiplication=Matrix(*)  SaturateOnIntegerOverflow=on  InputSameDT=on  OutDataTypeStr=Inherit: Same as first input
  I * w : Outport
  wires:
  Product/1 -> I * w/1
  Inertia_B/1 -> Product/1
  Omega_B/1 -> Product/2

== system M_6DoF_BS_Full_backup_11_25_2018/plant/Direction Cosine Matrix from quaternion/Subsystem/Subsystem ==
  p q r : Inport
  phi theta psi1 : Inport  Port=2
  Mux1 : Mux  Inputs=[3 3 3]
  Mux2 : Mux  Inputs=3
  phidot : Fcn  Expr=u[1]+(u[2]*u[4]+u[3]*u[7])*(u[5]/u[8])
  psidot : Fcn  Expr=(u[2]*u[4]+u[3]*u[7])/u[8]
  sincos : Trigonometry  Operator=sincos
  thetadot : Fcn  Expr=u[2]*u[7]-u[3]*u[4]
  phidot thetadot psi : Outport  InitialOutput=0
  wires:
  thetadot/1 -> Mux2/2
  psidot/1 -> Mux2/3
  phidot/1 -> Mux2/1
  sincos/2 -> Mux1/3
  sincos/1 -> Mux1/2
  phi theta psi1/1 -> sincos/1
  p q r/1 -> Mux1/1
  Mux2/1 -> phidot thetadot psi/1
  Mux1/1 -> psidot/1, phidot/1, thetadot/1

== matlab function M_6DoF_BS_Full_backup_11_25_2018/Attitude control/MATLAB Function ==
  data: t input; I_B input; I_r input; Tbar input; Gama1 input; Gama2 input; Omega_c input; W input; Omega input; Omega_ref input; Epsi input; Angles input; Angles_c input; Dot_Angles_c input; tau_x output; tau_y output; tau_z output; Omega_r input; Z1 output; Z2 output
function [tau_x,tau_y,tau_z,Z1,Z2] = fcn(t,I_B,I_r,Tbar,Gama1,Gama2,Omega_c,W,Omega,Omega_ref,Epsi,Angles,Angles_c,Dot_Angles_c,Omega_r)
%#codegen
% if t>=0.06
%     t
% end
%  t
Z1 = Angles - Angles_c;
Zbar1 = Z1-Epsi;
Z2 = Omega-Omega_c;

ez = [0;0;1];

M_B = cross(Omega,I_B*Omega);
M_Gyro = cross(Omega,ez)*I_r*Omega_r;

Tau = M_B+M_Gyro-I_B*Tbar*(Omega_c+W\Gama1*Z1)+I_B*Tbar*W\Dot_Angles_c...
-I_B*(W.'*Zbar1+Gama2*Z2);
tau_x = Tau(3);
tau_y = Tau(2);
tau_z = Tau(1);
end

== matlab function M_6DoF_BS_Full_backup_11_25_2018/MATLAB Function ==
  data: k input; w output; l input; b input; T input; tau_phi input; tau_theta input; tau_psi input; p output
function [w,p] = fcn(k,l,b,T,tau_phi,tau_theta,tau_psi)
%CALCULATE_RPM
%    [W1,W2,W3,W4] = CALCULATE_RPM(K,L,B,T,TAU_PHI,TAU_THETA,TAU_PSI)

%    This function was generated by the Symbolic Math Toolbox version 6.1.
%    27-Oct-2016 22:38:42

m=b;
n=k;
k=m;
b=n;

t2 = 1.0./b;
t3 = 1.0./k;
t4 = 1.0./l;
t5 = T.*b.*l;
t6 = k.*l.*tau_psi;
t7 = b.*tau_theta.*2.0;
w1 = sqrt(t2.*t3.*t4.*(t5+t6+t7).*(1.0./4.0));
t8 = b.*tau_phi.*2.0;
w2 = sqrt(t2.*t3.*t4.*(t5-t6+t8).*(1.0./4.0));
w3 = sqrt(t2.*t3.*t4.*(t5+t6-t7).*(1.0./4.0));
w4 = sqrt(t2.*t3.*t4.*(-t5+t6+t8).*(-1.0./4.0));
w = [w1;w2;w3;w4];

p=dot(b*w.^2,w);

end

== matlab function M_6DoF_BS_Full_backup_11_25_2018/Position control/MATLAB Function ==
  data: U input; m input; g input; Thurst_d output; EulerAngles input; theta_d output; phi_d output
function [Thurst_d,theta_d,phi_d] = fcn(U,m,g,EulerAngles) %#codegen


psi   = EulerAngles(1);
theta = EulerAngles(2);
phi   = EulerAngles(3);

U1 = U(1);
U2 = U(2);
U3 = U(3);
t2 = cos(psi);
t3 = sin(psi);
t4 = U3-g;
theta_d = atan((U1.*t2+U2.*t3)./t4);
phi_d = asin(-(U1.*t3-U2.*t2).*1.0./sqrt(U1.^2+U2.^2+t4.^2));
t5 = sin(phi);
t6 = cos(phi);
t7 = sin(theta);
Thurst_d = -m.*(U1.*(t3.*t5+t2.*t6.*t7)-U2.*(t2.*t5-t3.*t6.*t7)+t4.*t6.*cos(theta));

end

== matlab function M_6DoF_BS_Full_backup_11_25_2018/Reference Trajectory ==
  data: R_d output; V_d output; t input; psi output; rates_ref output; A_d output
function [R_d,V_d,psi,rates_ref,A_d] = fcn(t)
%#codegen

dt_1 = 20;
dt_2 = 60;
dt_3 = 20;
% tsum  = dt_1+dt_2+dt_3;

z_i_1 = 0;
z_f_1 = -20; 
zdot_i_1 = 0;
zdot_f_1 = 0;

z_i_2 = z_f_1;
z_f_2 = z_f_1; 
zdot_i_2 = 0;
zdot_f_2 = 0;

z_i_3 = z_f_2;
z_f_3 = z_i_1; 
zdot_i_3 = 0;
zdot_f_3 = 0;

rho = 1;
zeta1 = 1-0.5*(1+tanh((t-dt_1)/rho));
zeta2_l = 0.5*(1+tanh((t-dt_1)/rho));
zeta2_u = 1-0.5*(1+tanh((t-(dt_1+dt_2))/rho));
zeta2 = zeta2_l*zeta2_u;
zeta3 = 0.5*(1+tanh((t-(dt_1+dt_2))/rho));

[z1,zdot1]= CubicState(t,dt_1,z_i_1,z_f_1,zdot_i_1,zdot_f_1);
[z2,zdot2]= CubicState(t-dt_1,dt_2,z_i_2,z_f_2,zdot_i_2,zdot_f_2);
[z3,zdot3]= CubicState(t-(dt_1+dt_2),dt_3,z_i_3,z_f_3,zdot_i_3,zdot_f_3);
    
z    = zeta1*z1+zeta2*z2+zeta3*z3;
zdot = zeta1*zdot1+zeta2*zdot2+zeta3*zdot3;

%%

x_i_1 = 0;
x_f_1 = 100; 
xdot_i_1 = 0;
xdot_f_1 = 15;

x_i_2 = x_f_1;
x_f_2 = x_i_2+1.5*xdot_f_1*dt_2; 
xdot_i_2 = xdot_f_1;
xdot_f_2 = xdot_i_2;

x_i_3 = x_f_2;
x_f_3 = x_i_3+x_f_1; 
xdot_i_3 = xdot_f_1;
xdot_f_3 = 0;

rho = 1;
zeta1 = 1-0.5*(1+tanh((t-dt_1)/rho));
zeta2_l = 0.5*(1+tanh((t-dt_1)/rho));
zeta2_u = 1-0.5*(1+tanh((t-(dt_1+dt_2))/rho));
zeta2 = zeta2_l*zeta2_u;
zeta3 = 0.5*(1+tanh((t-(dt_1+dt_2))/rho));

[x1,xdot1]= CubicState(t,dt_1,x_i_1,x_f_1,xdot_i_1,xdot_f_1);
[x2,xdot2]= CubicState(t-dt_1,dt_2,x_i_2,x_f_2,xdot_i_2,xdot_f_2);
[x3,xdot3]= CubicState(t-(dt_1+dt_2),dt_3,x_i_3,x_f_3,xdot_i_3,xdot_f_3);

x    = zeta1*x1+zeta2*x2+zeta3*x3;
xdot = zeta1*xdot1+zeta2*xdot2+zeta3*xdot3;

    
y = 0;
ydot = 0;
    


R_d = [x;y;z];
V_d = [xdot;ydot;zdot];
A_d = [0;0;0];
psi = 0;
rates_ref = [0;0;0];

end

== matlab function M_6DoF_BS_Full_backup_11_25_2018/Attitude control/MATLAB Function1 ==
  data: Angles input; W output
function W = fcn(Angles) %#codegen
theta = Angles(2);
phi = Angles(3);

Sphi = sin(phi);
Cphi = cos(phi);
Tantheta = tan(theta);
Sectheta = sec(theta);
W = [1, Sphi*Tantheta, Cphi*Tantheta;
     0,          Cphi,         -Sphi;
     0, Sphi*Sectheta, Cphi*Sectheta];
end

== matlab function M_6DoF_BS_Full_backup_11_25_2018/Attitude control/MATLAB Function2 ==
  data: X input; Angles_c input; Xdot output; Lambda input
function Xdot = fcn(X,Angles_c,Lambda) %#codegen
Xdot = zeros(6,1);
X1 = X(1:3,1);
X2 = X(4:6,1);
Xdot(1:3,1) = X2;
Xdot(4:6,1) = -2*Lambda*X1-Lambda*Lambda*(X1-Angles_c);
end

== matlab function M_6DoF_BS_Full_backup_11_25_2018/Reference Trajectory1 ==
  data: R_d output; V_d output; t input; psi output; rates_ref output; tf_1 input; zf_1 input; tf_2 input; t_phase3 input; xdot_cruise input; deltaT input; A_d output
function [R_d,V_d,psi,rates_ref,A_d] = fcn(t,tf_1,zf_1,tf_2,t_phase3,xdot_cruise,deltaT)
%#codegen

% B: commenting on Ehsan's trajectory and defining a new one

a=xdot_cruise * 0;
% initial positions and rates
x = 0+a; 
y = 0; 
z = 0;
xdot = 0;
ydot = 0;
zdot = 0;
xddot = 0;
yddot = 0;
zddot = 0;


% tangential velocity for circular motion

R = 80;

vs = 2*pi*R / (tf_2 - tf_1 -deltaT) ;

ac_cruise = vs^2/R ;

om_cruise = vs / R ;

alp = om_cruise / deltaT ;

% take-off phase

if t<=tf_1
    
    % side velocity
    xdot = 0;
    ydot = 0;
    
    % target altitude and the time we hope to be there
    z_f = zf_1;
    tf = tf_1;
    
    a = -(2*z_f)/tf^3;
    b = (3*z_f)/tf^2;
    z = a*t.^3+b*t.^2;
    
    zdot = 3*a*t.^2+2*b*t;
    zddot = 6*a*t+2*b;
    
    %% cruise phase
    
elseif t>tf_1 && t<=tf_2
    
    z = zf_1;
    zdot = 0;
    
    % accelarating
    if (t-tf_1)<=deltaT
        
        t5 = t-tf_1;
        
        om = alp * t5 ;
        
        ac = R * om^2 ;
        
        theta = 1/2 * alp * t5^2 + pi ;
        
        xddot = - ac * cos(theta) - R * alp * sin(theta);
        
        yddot =  ac * sin(theta) - R * alp * cos(theta);
        
        xdot =  - R * om *  sin(theta) ;
        
        ydot =  - R * om * cos(theta) ;
                
        x = R * cos(theta) + R ;
        
        y =  -R * sin(theta) ;
        
        %         xddot_cruise = xdot_cruise/deltaT;
        %         xdot = xddot_cruise*(t-tf_1);
        %         x = 0.5*xddot_cruise*(t-tf_1)^2;
        
        % cruise with constant speed
        
    elseif (t-tf_1)>deltaT && (t-tf_1)<(tf_2-deltaT)
        
        t5 = t-tf_1-deltaT;
        t6 = deltaT;
        
        theta = om_cruise * t5 + pi + alp * deltaT^2 /2  ;
        
        xdot = - vs * sin(theta) ;
        ydot = - vs * cos(theta) ;
        
        xddot = - ac_cruise * cos(theta) ;
        yddot =  ac_cruise * sin(theta) ;

        x = R * cos(theta) + R ;    
        y =  -R * sin(theta) ;
        
        %         xdot = xdot_cruise;
        %         x = 0.5*xddot_cruise*deltaT^2 + xdot_cruise*(t-tf_1-deltaT);
        
    end
    % break and get ready to land
    
    if t>(tf_2-deltaT)
 
        tc = (tf_2-tf_1-2*deltaT);
        
        t5 = t-(tf_2-deltaT) ;
        
        % alp should be negative value od speed up
        
        om = om_cruise - alp * t5 ;
        
        ac = R * om^2 ;
        
        theta = om_cruise * tc + pi + 1/2 * alp * deltaT^2  - 1/2 * alp * t5^2 + om_cruise * t5;       
      
        xddot = - ac * cos(theta) - R * alp * sin(theta);
        yddot =  ac * sin(theta) - R * alp * cos(theta);
        
        xdot =  - R * om *  sin(theta) ;       
        ydot =  - R * om * cos(theta) ; 

        x = R * cos(theta) + R ;    
        y =  -R * sin(theta) ;
                 
        %        xdot = xdot_cruise-xdot_cruise/deltaT*(t-(tf_2-deltaT));
        %        x = 0.5*deltaT*xdot_cruise+xdot_cruise*(tf_2-tf_1-2*deltaT)+0.5*(xdot_cruise+xdot)*(t-(tf_2-deltaT));
    end
    
    %% landing phase
    
elseif t>tf_2
    
    x = 0;
    y = 0;
    xdot = 0;
    ydot =0;
    z_i = zf_1;
    tt = t-tf_2;
    tf = t_phase3;
    a = (2*z_i)/tf^3;
    b = -(3*z_i)/tf^2;
    d = z_i;
    z = a*tt.^3+b*tt.^2+d;
    zdot = 3*a*tt.^2+2*b*tt;
    
    %     x = deltaT*xdot_cruise+xdot_cruise*(tf_2-tf_1-2*deltaT);
    %     xdot = 0;
    %     z_i = zf_1;
    %     tt = t-tf_2;
    %     tf = t_phase3;
    %     a = (2*z_i)/tf^3;
    %     b = -(3*z_i)/tf^2;
    %     d = z_i;
    %     z = a*tt.^3+b*tt.^2+d;
    %     zdot = 3*a*tt.^2+2*b*tt;
    
end
R_d = [x;y;z];
V_d = [xdot;ydot;zdot];
A_d = [xddot;yddot;zddot];
psi = 0;
rates_ref = [0;0;0];

end

== matlab function M_6DoF_BS_Full_backup_11_25_2018/MATLAB Function2 ==
  settings: updateMethod=DISCRETE
  data: rpm_guesses input; RPM output; RPM2 output; V_rel_B input; angles input; t input; k input; b input; Tau_initial output; T_final output; Tau_final output; l input; geometry data_store_memory
function [RPM,RPM2,Tau_initial,T_final,Tau_final] = Radial_inflow(rpm_guesses,V_rel_B,angles,t,k,b,l)
%#codegen

% governing equations

% T=T1+T2+T3+T4 ;
% TA1=l*(T4-T2) ; roll positive right wing down
% TA2=l*(T1-T3) ; pitch up positive
% TA3=ta1+ta2+ta3+ta4 ;
% predefining vriables for Codegen

T_final=0;
Tau_initial=zeros(3,1);
Tau_final=zeros(3,1);
T2=zeros(4,1);

TA=zeros(3,1);
TA1=zeros(4,1);
TA2=zeros(4,1);
TA3=zeros(4,1);
ta1=zeros(4,1);
ta2=zeros(4,1);
ta3=zeros(4,1);

RPM2=zeros(4,1);
RPM=zeros(4,1);


T = b * rpm_guesses.^2;       % requested thrust from rotor r
Tau = k * rpm_guesses.^2;     % requested torques from rotor r


for i=1:4
    
    
    subfcn2 = @(rpm) inv_engine_new(rpm,V_rel_B,T(i));
    
    rpm=golden_search(100,20000,subfcn2);
    
    [~,~,yaw]=inv_engine_new(rpm,V_rel_B,T(i));
    
    % RPM to rad/second
    RPM(i)= rpm*2*pi/60;
    
    ta1(i) = 0;
    ta2(i) = 0;
    ta3(i) = yaw * (-1)^(i+1);
    
    
end

Tau_initial=[sum(ta1);sum(ta2);sum(ta3)];

% end of old way -- there is no control on TA3 that can make the system
% unstable, to do the new way only comment RPM(r) ane let the code keep
% running to the next section

%% new addition to help with yaw moment

% here we need to find a way to chage RPMs a bit such that they also
% provide the required Ta3. So, we can find the thrust and torque
% coefficients for a specific time and flight condition.

bb=T./RPM.^2;
kk=Tau./RPM.^2;

M=[bb'; ...
    0,bb(2)*l,0,-bb(4)*l;...
    bb(1)*l,0,-bb(3)*l,0;...
    kk(1),-kk(2),kk(3),-kk(4)];

T_tot=sum(T);

% we use the requsted thrust and torque - here we used the actual
% conventions, down pos z, right wing pos y, pointing to nose pos x

TA(1) = l* (T(2)-T(4)) - Tau_initial(1); % roll
TA(2) = l* (T(1)-T(3)) - Tau_initial(2); % pitch
TA(3) = dot([k,-k,k,-k],rpm_guesses.^2'); %yaw

% newly obtained RPMs
RPM2=(M\[T_tot;TA(1);TA(2);TA(3)]).^0.5;

% now let's see how much thrust and torque they make

for i=1:4
    % input to propeller code must be RPM not rev/sec
    [T,yaw,~]=Propeller(RPM2(i)*60/(2*pi),V_rel_B);
    
    T2(i)=T;
    TA1(i)=0;
    TA2(i)=0;
    TA3(i)=yaw* (-1)^(i+1);
    
end

TA_rotor=[sum(TA1);sum(TA2);sum(TA3)];

% here since we don't use negative thrusts, conventions are changed
T_final=sum(T2);
Tau_final(1,1)=l*(T2(2)-T2(4))+TA_rotor(1) ; % roll
Tau_final(2,1)=l*(T2(1)-T2(3))+TA_rotor(2) ; % pitch
Tau_final(3,1)=TA_rotor(3) ;

end

== matlab function M_6DoF_BS_Full_backup_11_25_2018/Aero models/MATLAB Function1 ==
  settings: updateMethod=DISCRETE
  data: RPM output; RPM2 output; rpm_guesses input; V_rel_B input; angles input; t input; k input; b input; Tau_initial output; T_final output; Tau_final output; l input; geometry data_store_memory; power output
%     Copyright (C) 12/12/2018  Regents of the University of Michigan
%     Aerospace Engineering Department
%     Computational Aeroscience Lab, written by Behdad Davoudi

%     This program is free software: you can redistribute it and/or modify
%     it under the terms of the GNU General Public License as published by
%     the Free Software Foundation, either version 3 of the License, or
%     (at your option) any later version.
% 
%     This program is distributed in the hope that it will be useful,
%     but WITHOUT ANY WARRANTY; without even the implied warranty of
%     MERCHANTABILITY or FITNESS FOR A PARTICULAR PURPOSE.  See the
%     GNU General Public License for more details.
% 
%     You should have received a copy of the GNU General Public License
%     along with this program.  If not, see <https://www.gnu.org/licenses/>.

function [RPM,RPM2,Tau_initial,T_final,Tau_final,power] = FWF(rpm_guesses,V_rel_B,angles,t,k,b,l)
%#codegen

% governing equations

% T=T1+T2+T3+T4 ;
% TA1=l*(T4-T2) ;   roll positive right wing down
% TA2=l*(T1-T3) ;    pitch up positive
% TA3=ta1+ta2+ta3+ta4 ;

% it looks like in atitude control output of the functin should be pitch
% down positive

%%
% predefining vriables for Codegen

T_final=0;
Tau_initial=zeros(3,1);
Tau_final=zeros(3,1);
T2=zeros(4,1);
pow=zeros(4,1);

TA=zeros(3,1);
TA1=zeros(4,1);
TA2=zeros(4,1);
TA3=zeros(4,1);
ta1=zeros(4,1);
ta2=zeros(4,1);
ta3=zeros(4,1);

RPM2=zeros(4,1);
RPM=zeros(4,1);

T = b * rpm_guesses.^2; % requested thrust from rotor r
Tau = k * rpm_guesses.^2;     % requested torques from rotor r

for i=1:4
    % optimization to find optimum rpm where both momentum annd blade element theories match
    
    subfcn2 = @(rpm) try1(rpm,V_rel_B,T(i));
    
    rpm=golden_search(100,16000,subfcn2);
    
    [~,roll,pitch,yaw]=try1(rpm,V_rel_B,T(i));
    
    % rpm to rad/second
    RPM(i)=rpm*2*pi/60;
    
    % torques of a rotor - rotor 1 is the leading edge rotor,left
    % number 2, right number 4, aft number, 1 and 3 ccw. 2 and 4 cw.
    
    heading=atan(V_rel_B(2)/(V_rel_B(1)+0.000001))
    ta1(i) = roll * cos(heading) * (-1)^(i+1) - pitch * sin(heading);
    ta2(i) = roll * sin(heading) * (-1)^(i+1) + pitch * cos(heading) ;
    % the sign will be taken care of in Matrix M -- no worries!
    ta3(i) = yaw * (+1)^(i+1);
    
end

Tau_initial=[sum(ta1);sum(ta2);sum(ta3)];

%% new addition to help with yaw moment

% here we need to find a way to change RPMs a bit such that they also
% provide the required Ta3. So, we can find the thrust and torque
% coefficients for a specific time and flight condition.

bb=T./RPM.^2;
kk=ta3./RPM.^2;

M=[bb'; ...
  0,bb(2)*l,0,-bb(4)*l;...
  bb(1)*l,0,-bb(3)*l,0;...
  kk(1),-kk(2),kk(3),-kk(4)];

T_tot=sum(T);

% we use the requsted thrust and torque - here we used the actual
% conventions, down pos z, right wing pos y, pointing to nose pos x

TA(1) = l* (T(2)-T(4)) - Tau_initial(1); % roll
TA(2) = l* (T(1)-T(3)) - Tau_initial(2); % pitch
TA(3) = dot([k,-k,k,-k],rpm_guesses.^2'); % yaw

% newly obtained RPMs
RPM2=(M\[T_tot;TA(1);TA(2);TA(3)]).^0.5;

% now let's see how much thrust and torque they make

for i=1:4
    % input to propeller code must be RPM not rev/sec
    
    subfcn2 = @(T) try2(T,rpm,V_rel_B);
    
    T=golden_search(0,20,subfcn2);
    
    [~,roll,pitch,yaw,T]=try2(T,RPM2(i)*60/(2*pi),V_rel_B);
    pow(i)=yaw * RPM2(i);
    T2(i)=T;
    heading=atan(V_rel_B(2)/(V_rel_B(1)+0.000001));
    TA1(i) = roll * cos(heading) * (-1)^(i+1) - pitch * sin(heading);
    TA2(i) = roll * sin(heading) * (-1)^(i+1) + pitch * cos(heading) ;
    TA3(i)=yaw* (-1)^(i+1);

end

TA_rotor=[sum(TA1);sum(TA2);sum(TA3)];

% here since we don't use negative thrusts, conventions are changed
T_final=sum(T2);
Tau_final(1,1)=l*(T2(2)-T2(4))+TA_rotor(1) ; % roll
Tau_final(2,1)=l*(T2(1)-T2(3))+TA_rotor(2) ; % pitch
Tau_final(3,1)=TA_rotor(3) ;
power = sum(pow) ;

end
